simulink model "static_attitude_sim"  (R2021b)
settings: Solver=VariableStepAuto  StartTime=0.0  StopTime=10.0  RelTol=1e-3
values from neighbouring files (symbols this model uses):
  stdDev = [0.1 0.15 0.2 0.1 0.05 0.15 0.25 0.1 0.2 0.05]    [static_attitude_var.m]
libraries: STATIC_ATT_DET x3, kinematic_transform x3, ERRORS x2
settings Model: Creator=Davide  LastModifiedBy=Davide

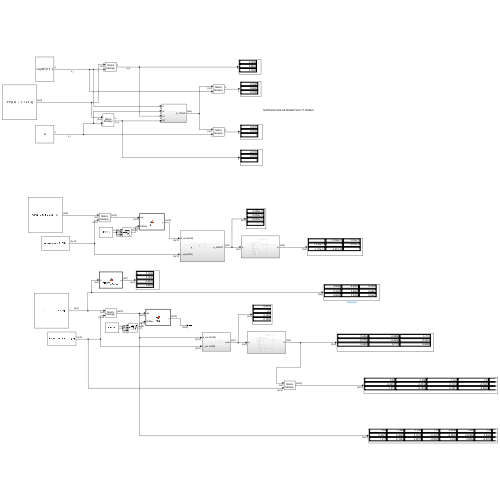
[thumbnail: Simulink's stored preview of the top-level diagram]
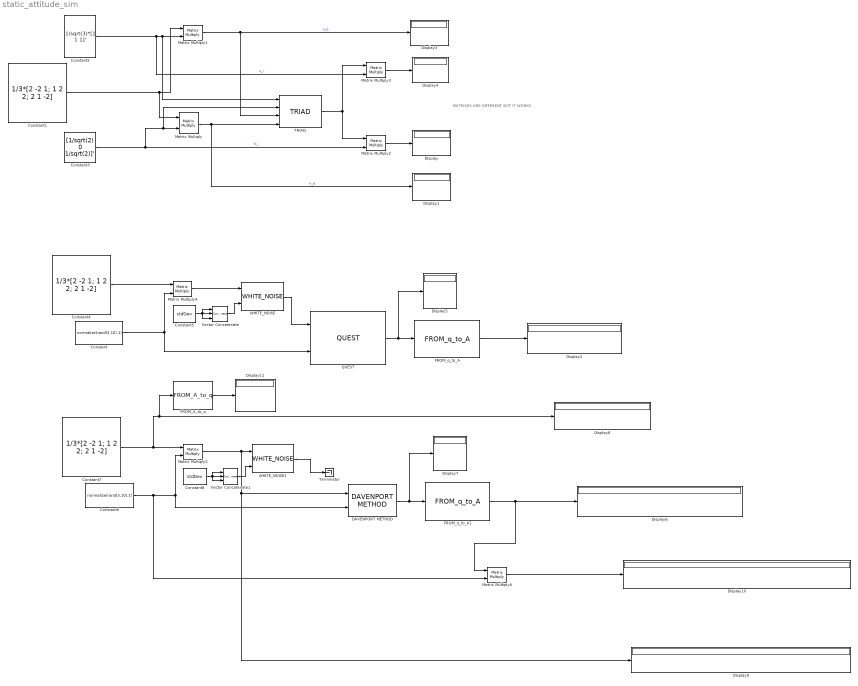
== system static_attitude_sim ==
  note: MATRIXES ARE DIFFERENT BUT IT WORKS
  Constant : Constant  Value=normalize(rand(3,10),1)
  Constant1 : Constant  Value=1/3*[2 -2 1; 1 2 2; 2 1 -2]
  Constant2 : Constant  Value=1/sqrt(3)*[1 1 1]'
  Constant3 : Constant  Value=[1/sqrt(2) 0 1/sqrt(2)]'
  Constant4 : Constant  Value=1/3*[2 -2 1; 1 2 2; 2 1 -2]
  Constant5 : Constant  Value=stdDev  VectorParams1D=off
  Constant6 : Constant  Value=normalize(rand(3,10),1)
  Constant7 : Constant  Value=1/3*[2 -2 1; 1 2 2; 2 1 -2]
  Constant8 : Constant  Value=stdDev  VectorParams1D=off
  DAVENPORT METHOD : STATIC_ATT_DET/DAVENPORT METHOD  SystemSampleTime=-1  VariantActivationTime=update diagram  Latency=0  AutoFrameSizeCalculation=off
      settings: SourceProductName=Attitude Determination (static)
  Display{,1..11} (12 alike) : Display
  FROM_A_to_q : kinematic_transform/FROM_A_to_q  SystemSampleTime=-1  VariantActivationTime=update diagram  Latency=0  AutoFrameSizeCalculation=off
      settings: SourceProductName=Kinematic Transformation
  FROM_q_to_A : kinematic_transform/FROM_q_to_A  SystemSampleTime=-1  VariantActivationTime=update diagram  Latency=0  AutoFrameSizeCalculation=off
      settings: SourceProductName=Kinematic Transformation
  FROM_q_to_A1 : kinematic_transform/FROM_q_to_A  SystemSampleTime=-1  VariantActivationTime=update diagram  Latency=0  AutoFrameSizeCalculation=off
      settings: SourceProductName=Kinematic Transformation
  Matrix Multiply{,1..6} (7 alike) : Product  Multiplication=Matrix(*)
  QUEST : STATIC_ATT_DET/QUEST  SystemSampleTime=-1  VariantActivationTime=update diagram  Latency=0  AutoFrameSizeCalculation=off
      settings: SourceProductName=Attitude Determination (static)
  TRIAD : STATIC_ATT_DET/TRIAD  SystemSampleTime=-1  VariantActivationTime=update diagram  Latency=0  AutoFrameSizeCalculation=off
      settings: SourceProductName=Attitude Determination (static)
  Terminator : Terminator
  Vector Concatenate : Concatenate  NumInputs=3  Mode=Multidimensional array
  Vector Concatenate1 : Concatenate  NumInputs=3  Mode=Multidimensional array
  WHITE_NOISE : ERRORS/WHITE_NOISE  SystemSampleTime=-1  VariantActivationTime=update diagram  Latency=0  AutoFrameSizeCalculation=off
      settings: SourceProductName=Errors
  WHITE_NOISE1 : ERRORS/WHITE_NOISE  SystemSampleTime=-1  VariantActivationTime=update diagram  Latency=0  AutoFrameSizeCalculation=off
      settings: SourceProductName=Errors
  wires:
  Matrix Multiply3/1 -> Display4/1
  Matrix Multiply2/1 -> Display/1
  TRIAD/1 -> Matrix Multiply3/1, Matrix Multiply2/1
  Matrix Multiply1/1 -> TRIAD/3, Display3/1  "s_b"
  Constant1/1 -> Matrix Multiply/1, Matrix Multiply1/1
  Constant2/1 -> TRIAD/1, Matrix Multiply1/2, Matrix Multiply3/2  "s_i"
  Matrix Multiply/1 -> TRIAD/4, Display1/1  "h_b"
  Constant3/1 -> Matrix Multiply2/2, TRIAD/2, Matrix Multiply/2  "h_i"
  Constant/1 -> Matrix Multiply4/2, QUEST/2
  Constant4/1 -> Matrix Multiply4/1
  Matrix Multiply4/1 -> WHITE_NOISE/1
  QUEST/1 -> Display5/1, FROM_q_to_A/1
  FROM_q_to_A/1 -> Display2/1
  Constant5/1 -> Vector Concatenate/3, Vector Concatenate/2, Vector Concatenate/1
  WHITE_NOISE/1 -> QUEST/1
  Vector Concatenate/1 -> WHITE_NOISE/2
  WHITE_NOISE1/1 -> Terminator/1
  Constant8/1 -> Vector Concatenate1/3, Vector Concatenate1/2, Vector Concatenate1/1
  Vector Concatenate1/1 -> WHITE_NOISE1/2
  DAVENPORT METHOD/1 -> Display7/1, FROM_q_to_A1/1
  FROM_q_to_A1/1 -> Matrix Multiply6/1, Display6/1
  Constant6/1 -> Matrix Multiply6/2, DAVENPORT METHOD/2, Matrix Multiply5/2
  Constant7/1 -> FROM_A_to_q/1, Display8/1, Matrix Multiply5/1
  Matrix Multiply5/1 -> DAVENPORT METHOD/1, Display9/1, WHITE_NOISE1/1
  Matrix Multiply6/1 -> Display10/1
  FROM_A_to_q/1 -> Display11/1
